simulink library "Cassie_CommandBlock_Library_5"  (R2017b)
settings: Solver=VariableStepAuto  StartTime=0.0  StopTime=10.0  RelTol=1e-3
undefined symbols (not defined in the file): dq, DynamicMatrixLibrary, isSim, q, sample_time
libraries: slrtlib x125, Cassie_CommandBlock_Library_3 x1
(part 1 of 3)
settings Model: Creator=81068  LastModifiedBy=81068

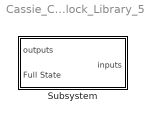
== system Cassie_CommandBlock_Library_5 ==
  Subsystem : Subsystem

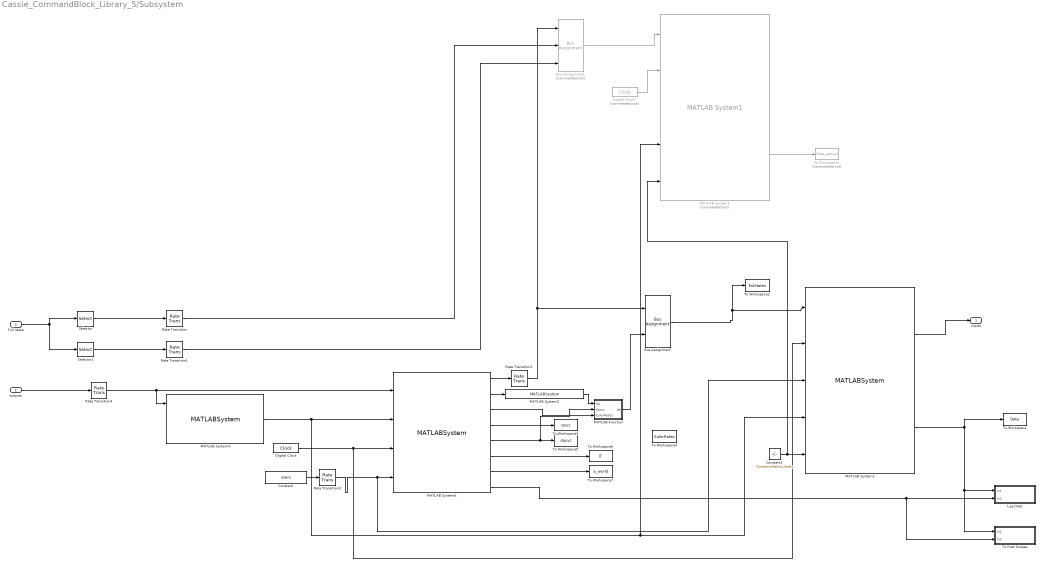
== system Cassie_CommandBlock_Library_5/Subsystem ==
  outputs : Inport  OutDataTypeStr=Bus: CassieOutBus
  Full State : Inport  Port=2
  Bus Assignment : BusAssignment  AssignedSignals=dq
  Bus Assignment1 : BusAssignment  Commented=on  AssignedSignals=q,dq
  Constant : Constant  Value=isSim  OutDataTypeStr=int8  LockScale=on
  Constant1 : Constant  Value=DynamicMatrixLibrary  OutDataTypeStr=Bus: cassieDynamicMatrixLibraryBus
  Digital Clock : DigitalClock  SampleTime=sample_time
  Digital Clock1 : DigitalClock  Commented=on  SampleTime=sample_time
  "Log Data " : Subsystem
  MATLAB Function : MATLAB Function  TreatAsAtomicUnit=on
  MATLAB System1 : MATLABSystem  System=Cassie_Controller_3  Kp_pitch=c_Kp_pitch  Kd_pitch=c_Kd_pitch  Kp_roll=c_Kp_roll  Kd_roll=c_Kd_roll  Kp_yaw=c_Kp_yaw  Kd_yaw=c_Kd_yaw  Kp_abduction=c_Kp_abduction  Kp_rotation=c_Kp_rotation  Kp_thigh=c_Kp_thigh  Kp_knee=c_Kp_knee  Kp_toe=c_Kp_toe  Kd_abduction=c_Kd_abduction  Kd_rotation=c_Kd_rotation  Kd_thigh=c_Kd_thigh  Kd_knee=c_Kd_knee  Kd_toe=c_Kd_toe  Kp_st_rotation=c_Kp_st_rotation  Kd_st_rotation=c_Kd_st_rotation  u_abduction_swing_cp=c_u_abduction_swing_cp  u_roll_cp=c_u_roll_cp  u_pitch_cp=c_u_pitch_cp  u_knee_cp=c_u_knee_cp  CovPos_abduction=c_CovPos_abduction  CovPos_rotation=c_CovPos_rotation  CovPos_thigh=c_CovPos_thigh  CovPos_knee=c_CovPos_knee  CovPos_toe=c_CovPos_toe  CovPos_qj1=c_CovPos_qj1  CovPos_qj2=c_CovPos_qj2  CovPos_qj3=c_CovPos_qj3  CovVel_abduction=c_CovVel_abduction  CovVel_rotation=c_CovVel_rotation  CovVel_thigh=c_CovVel_thigh  CovVel_knee=c_CovVel_knee  CovVel_toe=c_CovVel_toe  CovVel_qj1=c_CovVel_qj1  CovVel_qj2=c_CovVel_qj2  CovVel_qj3=c_CovVel_qj3  Cov_Euler=c_Cov_Euler  Cov_Euler_rates=c_Cov_Euler_rates  Cov_Lx_LRToe_stTD0=c_Cov_Lx_LRToe_stTD0  Cov_Ly_LRToe_stTD0=c_Cov_Ly_LRToe_stTD0  Cov_rpx_LRToe_stTD0=c_Cov_rpx_LRToe_stTD0  Cov_rpy_LRToe_stTD0=c_Cov_rpy_LRToe_stTD0  torque_transition_time=c_torque_transition_time  knee_cp_time=c_knee_cp_time  st_rotation_torque_ramp_time=c_st_rotation_torque_ramp_time  com_x_offset=c_com_x_offset  Vx_tgd_offset=c_Vx_tgd_offset  Vy_tgd_offset=c_Vy_tgd_offset  stance_thre_lb=c_stance_thre_lb  stance_thre_ub=c_stance_thre_ub  stance_thre_lb_2=c_stance_thre_lb_2  stance_thre_ub_2=c_stance_thre_ub_2  IK_max_iter_num=c_IK_max_iter_num  yaw_error_fil_param=c_yaw_error_fil_param  rp_LRToe_fil_param=c_rp_LRToe_fil_param  adjusted_desired_roll_angle_fil_param=c_adjusted_desired_roll_angle_fil_param  use_dq_AR_for_PD=c_use_dq_AR_for_PD  lateral_correction_gain=c_lateral_correction_gain  one_step_max_vel_gain=c_one_step_max_vel_gain  max_st_rotation_motor_torque=c_max_st_rotation_motor_torque  KsL_1=c_KsL_1  KsL_2=c_KsL_2  KsR_1=c_KsR_1  KsR_2=c_KsR_2  toe_leave_ground_lb=c_toe_leave_ground_lb  toe_leave_ground_ub=c_toe_leave_ground_ub  sample_time=sample_time  SimulateUsing=Interpreted execution
      mask Type: Cassie_Controller_3
      mask Display:
      | disp('Cassie_Controller_3');
      | port_label('input',1,'EstStates');
      | port_label('input',2,'t_total');
      | port_label('input',3,'isSim');
      | port_label('input',4,'IRC');
      | port_label('input',5,'DynamicMatrixLibrary');
      | port_label('output',1,'userInputs');
      | port_label('output',2,'Data');
  MATLAB System2 : MATLABSystem  System=PolyRegressionFilter_2  sample_time=sample_time  history_length=c_history_length  dop=c_dop  signal_dim=20  delay=0  max_history_length=20  max_dop=3  SimulateUsing=Code generation
      mask Type: PolyRegressionFilter_2
      mask Display:
      | disp('PolyRegressionFilter_2');
      | port_label('input',1,'q');
      | port_label('output',1,'dq');
  MATLAB System3 : Cassie_CommandBlock_Library_3/Subsystem/MATLAB System1  Commented=on  Kp_pitch=c_Kp_pitch  Kd_pitch=c_Kd_pitch  Kp_roll=c_Kp_roll  Kd_roll=c_Kd_roll  Kp_yaw=c_Kp_yaw  Kd_yaw=c_Kd_yaw  Kp_abduction=c_Kp_abduction  Kp_rotation=c_Kp_rotation  Kp_thigh=c_Kp_thigh  Kp_knee=c_Kp_knee  Kp_toe=c_Kp_toe  Kd_abduction=c_Kd_abduction  Kd_rotation=c_Kd_rotation  Kd_thigh=c_Kd_thigh  Kd_knee=c_Kd_knee  Kd_toe=c_Kd_toe  Kp_st_rotation=c_Kp_st_rotation  Kd_st_rotation=c_Kd_st_rotation  u_abduction_swing_cp=c_u_abduction_swing_cp  u_roll_cp=c_u_roll_cp  u_pitch_cp=c_u_pitch_cp  u_knee_cp=c_u_knee_cp  CovPos_abduction=c_CovPos_abduction  CovPos_rotation=c_CovPos_rotation  CovPos_thigh=c_CovPos_thigh  CovPos_knee=c_CovPos_knee  CovPos_toe=c_CovPos_toe  CovPos_qj1=c_CovPos_qj1  CovPos_qj2=c_CovPos_qj2  CovPos_qj3=c_CovPos_qj3  CovVel_abduction=c_CovVel_abduction  CovVel_rotation=c_CovVel_rotation  CovVel_thigh=c_CovVel_thigh  CovVel_knee=c_CovVel_knee  CovVel_toe=c_CovVel_toe  CovVel_qj1=c_CovVel_qj1  CovVel_qj2=c_CovVel_qj2  CovVel_qj3=c_CovVel_qj3  Cov_Euler=c_Cov_Euler  Cov_Euler_rates=c_Cov_Euler_rates  Cov_Lx_LRToe_stTD0=c_Cov_Lx_LRToe_stTD0  Cov_Ly_LRToe_stTD0=c_Cov_Ly_LRToe_stTD0  Cov_rpx_LRToe_stTD0=c_Cov_rpx_LRToe_stTD0  Cov_rpy_LRToe_stTD0=c_Cov_rpy_LRToe_stTD0  torque_transition_time=c_torque_transition_time  knee_cp_time=c_knee_cp_time  st_rotation_torque_ramp_time=c_st_rotation_torque_ramp_time  com_x_offset=c_com_x_offset  Vx_tgd_offset=c_Vx_tgd_offset  Vy_tgd_offset=c_Vy_tgd_offset  stance_thre_lb=c_stance_thre_lb  stance_thre_ub=c_stance_thre_ub  stance_thre_lb_2=c_stance_thre_lb_2  stance_thre_ub_2=c_stance_thre_ub_2  IK_max_iter_num=c_IK_max_iter_num  yaw_error_fil_param=c_yaw_error_fil_param  rp_LRToe_fil_param=c_rp_LRToe_fil_param  adjusted_desired_roll_angle_fil_param=c_adjusted_desired_roll_angle_fil_param  use_dq_AR_for_PD=c_use_dq_AR_for_PD  lateral_correction_gain=c_lateral_correction_gain  one_step_max_vel_gain=c_one_step_max_vel_gain  max_st_rotation_motor_torque=c_max_st_rotation_motor_torque  KsL_1=c_KsL_1  KsL_2=c_KsL_2  KsR_1=c_KsR_1  KsR_2=c_KsR_2  toe_leave_ground_lb=c_toe_leave_ground_lb  toe_leave_ground_ub=c_toe_leave_ground_ub  sample_time=sample_time  SimulateUsing=Code generation
  MATLAB System4 : MATLABSystem  System=RadioCommandInterpreter  max_turn_per_sec=c_max_turn_per_sec  Vx_tgd_fil_param=c_Vx_tgd_fil_param  Vy_tgd_avg_fil_param=c_Vy_tgd_avg_fil_param  H_fil_param=c_H_fil_param  desired_com2stToe_lateral_fil_param=c_desired_com2stToe_lateral_fil_param  sample_time=sample_time  SimulateUsing=Code generation
      mask Type: RadioCommandInterpreter
      mask Display:
      | disp('RadioCommandInterpreter');
      | port_label('input',1,'cassieOutputs');
      | port_label('input',2,'t_total');
      | port_label('input',3,'isSim');
      | port_label('output',1,'IRC');
  MATLAB System6 : MATLABSystem  System=StateEstimator_3  CovPos_abduction=c_CovPos_abduction  CovPos_rotation=c_CovPos_rotation  CovPos_thigh=c_CovPos_thigh  CovPos_knee=c_CovPos_knee  CovPos_toe=c_CovPos_toe  CovPos_qj1=c_CovPos_qj1  CovPos_qj2=c_CovPos_qj2  CovPos_qj3=c_CovPos_qj3  Cov_Euler=c_Cov_Euler  Cov_LinearAccelerator_xy=c_Cov_LinearAccelerator_xy  Cov_LinearAccelerator_z=c_Cov_LinearAccelerator_z  Cov_rpx_LRToe_body=c_Cov_rpx_LRToe_body  Cov_rpy_LRToe_body=c_Cov_rpy_LRToe_body  Cov_rpz_LRToe_body=c_Cov_rpz_LRToe_body  vx_slide_toe_1=c_vx_slide_toe_1  vx_slide_toe_2=c_vx_slide_toe_2  Tx_slide_toe_2=c_Tx_slide_toe_2  vy_slide_toe_1=c_vy_slide_toe_1  vy_slide_toe_2=c_vy_slide_toe_2  Ty_slide_toe_2=c_Ty_slide_toe_2  vz_slide_toe_1=c_vz_slide_toe_1  vz_slide_toe_2=c_vz_slide_toe_2  Tz_slide_toe_2=c_Tz_slide_toe_2  KsL_1=c_KsL_1  KsL_2=c_KsL_2  KsR_1=c_KsR_1  KsR_2=c_KsR_2  sample_time=sample_time  SimulateUsing=Code generation
      mask Type: StateEstimator_3
      mask Display:
      | disp('StateEstimator_3');
      | port_label('input',1,'cassieOutputs');
      | port_label('input',2,'IRC');
      | port_label('input',3,'t_total');
      | port_label('input',4,'isSim');
      | port_label('output',1,'EstStates');
      | port_label('output',2,'q');
      | port_label('output',3,'EulerRates');
      | port_label('output',4,'qxyz');
      | port_label('output',5,'dqxyz');
      | port_label('output',6,'IT');
      | port_label('output',7,'a_world');
      | port_label('output',8,'StateEstimator_Data');
  Rate Transition{,1..4} (5 alike) : RateTransition  OutPortSampleTime=sample_time
  Selector : Selector  InputPortWidth=40  IndexOptions=Index vector (dialog)  Indices=1:20  OutputSizes=1
  Selector1 : Selector  InputPortWidth=40  IndexOptions=Index vector (dialog)  Indices=21:40  OutputSizes=1
  "To Host Scopes " : Subsystem
  To Workspace : ToWorkspace  VariableName=Data  SaveFormat=Timeseries  SampleTime=-1
  To Workspace1 : ToWorkspace  Commented=on  VariableName=Data_perfect  SaveFormat=Timeseries  SampleTime=-1
  To Workspace2 : ToWorkspace  VariableName=EstStates  SaveFormat=Timeseries  SampleTime=-1
  To Workspace3 : ToWorkspace  VariableName=EulerRates  SaveFormat=Timeseries  SampleTime=-1
  To Workspace4 : ToWorkspace  VariableName=qxyz  SaveFormat=Timeseries  SampleTime=-1
  To Workspace5 : ToWorkspace  VariableName=dqxyz  SaveFormat=Timeseries  SampleTime=-1
  To Workspace6 : ToWorkspace  VariableName=IT  SaveFormat=Timeseries  SampleTime=-1
  To Workspace7 : ToWorkspace  VariableName=a_world  SaveFormat=Timeseries  SampleTime=-1
  "inputs " : Outport
  wires:
  outputs/1 -> Rate Transition4/1
  MATLAB System1/2 -> "Log Data "/1(In1), "To Host Scopes "/1(In1), To Workspace/1
  Digital Clock/1 -> MATLAB System6/3, MATLAB System1/2
  Constant/1 -> Rate Transition3/1
  MATLAB System6/1 -> Rate Transition2/1
  Full State/1 -> Selector1/1, Selector/1
  Selector/1 -> Rate Transition/1
  Selector1/1 -> Rate Transition1/1
  Rate Transition2/1 -> Bus Assignment/1, Bus Assignment1/1
  Rate Transition4/1 -> MATLAB System6/1, MATLAB System4/1
  Bus Assignment1/1 -> MATLAB System3/1
  Digital Clock1/1 -> MATLAB System3/2
  Rate Transition/1 -> Bus Assignment1/2
  Rate Transition1/1 -> Bus Assignment1/3
  MATLAB System3/2 -> To Workspace1/1
  Bus Assignment/1 -> To Workspace2/1, MATLAB System1/1
  MATLAB System1/1 -> "inputs "/1
  MATLAB System2/1 -> MATLAB Function/1("dq ")
  MATLAB Function/1(dq) -> Bus Assignment/2
  MATLAB System4/1 -> MATLAB System6/2, MATLAB System3/4, MATLAB System1/4
  Rate Transition3/1 -> MATLAB System1/3, MATLAB System6/4
  Constant1/1 -> MATLAB System3/5, MATLAB System1/5
  MATLAB System6/8 -> "To Host Scopes "/2(In2), "Log Data "/2(In2)
  MATLAB System6/7 -> To Workspace7/1
  MATLAB System6/6 -> To Workspace6/1
  MATLAB System6/5 -> MATLAB Function/2(dqxyz), To Workspace5/1
  MATLAB System6/2 -> MATLAB System2/1
  MATLAB System6/3 -> MATLAB Function/3(EulerRates)
  MATLAB System6/4 -> To Workspace4/1

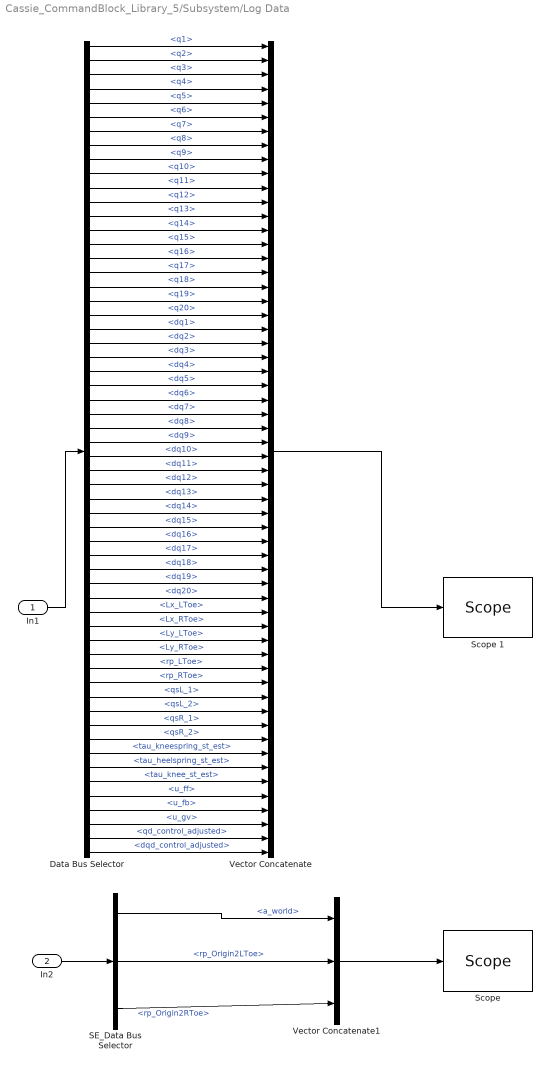
== system Cassie_CommandBlock_Library_5/Subsystem/Log Data  ==
  In1 : Inport  OutDataTypeStr=Bus: cassieDataBus
  In2 : Inport  Port=2  OutDataTypeStr=Bus: StateEstimator_DataBus
  Data Bus Selector : BusSelector  OutputSignals=q1,q2,q3,q4,q5,q6,q7,q8,q9,q10,q11,q12,q13,q14,q15,q16,q17,q18,q19,q20,dq1,dq2,dq3,dq4,dq5,dq6,dq7,dq8,dq9,dq10,dq11,dq12,dq13,dq14,dq15,dq16,dq17,dq18,dq19,dq20,Lx_LToe,Lx_RToe,Ly_LToe,Ly_RToe,rp_LToe,rp_RToe,qsL_1,qsL_2,qsR_1,qsR_2,tau_kneespring_st_est,tau_heelspring_st_est,tau_knee_st_est,u_ff,u_fb,u_gv,qd_control_adjusted,dqd_control_adjusted
  SE_Data Bus Selector : BusSelector  OutputSignals=a_world,rp_Origin2LToe,rp_Origin2RToe
  "Scope " : slrtlib/Displays and Logging/Scope   scopeno=6  scopetype=File  autostart=on  viewmode=Graphical redraw  formatstr='%15.6f'  grid=on  ylimits=[0,0]  nosamples=250  noprepostsamples=0  interleave=1  triggermode=FreeRun  triggersignal=1  trigsignalfromport=off  triggerlevel=0.0  triggerslope=Either  triggerscope=1  triggersample=0  filename=SE_DATA.dat  mode=Lazy  writesize=512*8  autorestart=on  dynamicfilemode=off  maxwritefilesize=4*1024^3
  Scope 1 : slrtlib/Displays and Logging/Scope   scopeno=5  scopetype=File  autostart=on  viewmode=Graphical redraw  formatstr='%15.6f'  grid=on  ylimits=[0,0]  nosamples=250  noprepostsamples=0  interleave=1  triggermode=FreeRun  triggersignal=1  trigsignalfromport=off  triggerlevel=0.0  triggerslope=Either  triggerscope=1  triggersample=0  filename=DATA.dat  mode=Lazy  writesize=512*8  autorestart=on  dynamicfilemode=off  maxwritefilesize=4*1024^3
  Vector Concatenate : Concatenate  NumInputs=58
  Vector Concatenate1 : Concatenate  NumInputs=3
  wires:
  In1/1 -> Data Bus Selector/1
  In2/1 -> SE_Data Bus Selector/1
  SE_Data Bus Selector/1 -> Vector Concatenate1/1  "<a_world>"
  SE_Data Bus Selector/2 -> Vector Concatenate1/2  "<rp_Origin2LToe>"
  SE_Data Bus Selector/3 -> Vector Concatenate1/3  "<rp_Origin2RToe>"
  Vector Concatenate1/1 -> "Scope "/1
  Vector Concatenate/1 -> Scope 1/1
  Data Bus Selector/1 -> Vector Concatenate/1  "<q1>"
  Data Bus Selector/2 -> Vector Concatenate/2  "<q2>"
  Data Bus Selector/3 -> Vector Concatenate/3  "<q3>"
  Data Bus Selector/4 -> Vector Concatenate/4  "<q4>"
  Data Bus Selector/5 -> Vector Concatenate/5  "<q5>"
  Data Bus Selector/6 -> Vector Concatenate/6  "<q6>"
  Data Bus Selector/7 -> Vector Concatenate/7  "<q7>"
  Data Bus Selector/8 -> Vector Concatenate/8  "<q8>"
  Data Bus Selector/9 -> Vector Concatenate/9  "<q9>"
  Data Bus Selector/10 -> Vector Concatenate/10  "<q10>"
  Data Bus Selector/11 -> Vector Concatenate/11  "<q11>"
  Data Bus Selector/12 -> Vector Concatenate/12  "<q12>"
  Data Bus Selector/13 -> Vector Concatenate/13  "<q13>"
  Data Bus Selector/14 -> Vector Concatenate/14  "<q14>"
  Data Bus Selector/15 -> Vector Concatenate/15  "<q15>"
  Data Bus Selector/16 -> Vector Concatenate/16  "<q16>"
  Data Bus Selector/17 -> Vector Concatenate/17  "<q17>"
  Data Bus Selector/18 -> Vector Concatenate/18  "<q18>"
  Data Bus Selector/19 -> Vector Concatenate/19  "<q19>"
  Data Bus Selector/20 -> Vector Concatenate/20  "<q20>"
  Data Bus Selector/21 -> Vector Concatenate/21  "<dq1>"
  Data Bus Selector/22 -> Vector Concatenate/22  "<dq2>"
  Data Bus Selector/23 -> Vector Concatenate/23  "<dq3>"
  Data Bus Selector/24 -> Vector Concatenate/24  "<dq4>"
  Data Bus Selector/25 -> Vector Concatenate/25  "<dq5>"
  Data Bus Selector/26 -> Vector Concatenate/26  "<dq6>"
  Data Bus Selector/27 -> Vector Concatenate/27  "<dq7>"
  Data Bus Selector/28 -> Vector Concatenate/28  "<dq8>"
  Data Bus Selector/29 -> Vector Concatenate/29  "<dq9>"
  Data Bus Selector/30 -> Vector Concatenate/30  "<dq10>"
  Data Bus Selector/31 -> Vector Concatenate/31  "<dq11>"
  Data Bus Selector/32 -> Vector Concatenate/32  "<dq12>"
  Data Bus Selector/33 -> Vector Concatenate/33  "<dq13>"
  Data Bus Selector/34 -> Vector Concatenate/34  "<dq14>"
  Data Bus Selector/35 -> Vector Concatenate/35  "<dq15>"
  Data Bus Selector/36 -> Vector Concatenate/36  "<dq16>"
  Data Bus Selector/37 -> Vector Concatenate/37  "<dq17>"
  Data Bus Selector/38 -> Vector Concatenate/38  "<dq18>"
  Data Bus Selector/39 -> Vector Concatenate/39  "<dq19>"
  Data Bus Selector/40 -> Vector Concatenate/40  "<dq20>"
  Data Bus Selector/41 -> Vector Concatenate/41  "<Lx_LToe>"
  Data Bus Selector/42 -> Vector Concatenate/42  "<Lx_RToe>"
  Data Bus Selector/43 -> Vector Concatenate/43  "<Ly_LToe>"
  Data Bus Selector/44 -> Vector Concatenate/44  "<Ly_RToe>"
  Data Bus Selector/45 -> Vector Concatenate/45  "<rp_LToe>"
  Data Bus Selector/46 -> Vector Concatenate/46  "<rp_RToe>"
  Data Bus Selector/47 -> Vector Concatenate/47  "<qsL_1>"
  Data Bus Selector/48 -> Vector Concatenate/48  "<qsL_2>"
  Data Bus Selector/49 -> Vector Concatenate/49  "<qsR_1>"
  Data Bus Selector/50 -> Vector Concatenate/50  "<qsR_2>"
  Data Bus Selector/51 -> Vector Concatenate/51  "<tau_kneespring_st_est>"
  Data Bus Selector/52 -> Vector Concatenate/52  "<tau_heelspring_st_est>"
  Data Bus Selector/53 -> Vector Concatenate/53  "<tau_knee_st_est>"
  Data Bus Selector/54 -> Vector Concatenate/54  "<u_ff>"
  Data Bus Selector/55 -> Vector Concatenate/55  "<u_fb>"
  Data Bus Selector/56 -> Vector Concatenate/56  "<u_gv>"
  Data Bus Selector/57 -> Vector Concatenate/57  "<qd_control_adjusted>"
  Data Bus Selector/58 -> Vector Concatenate/58  "<dqd_control_adjusted>"
